simulink model "rct_CSTR_OL"  (R2022a)
settings: Solver=ode45  StartTime=0  StopTime=10  RelTol=1e-3  EnableMultiTasking=on
settings Model: Creator=The MathWorks, Inc.  LastModifiedBy=The MathWorks, Inc.
settings SolverCC: AlgebraicLoopSolver=TrustRegion  MaxZcPerStep=1
settings DataIOCC: InitialState=[311.267; 8.5695]  LimitDataPoints=on  SaveFormat=Array  ReturnWorkspaceOutputs=off  SignalLoggingName=logsOut
settings OptimizationCC: BooleanDataType=off  DefaultParameterBehavior=Inlined  InlineInvariantSignals=on  BufferReuse=off  ExpressionDepthLimit=2147483647  InitFltsAndDblsToZero=on  LifeSpan=inf
settings DebuggingCC: SaveWithParameterizedLinksMsg=none  UnderspecifiedInitializationDetection=Classic  MergeDetectMultiDrivingBlocksExec=none  CheckExecutionContextPreStartOutputMsg=on  SignalResolutionControl=TryResolveAllWithWarning  MultiTaskDSMMsg=warning  MultiTaskCondExecSysMsg=none  UnconnectedInputMsg=warning  UnconnectedOutputMsg=warning  UnconnectedLineMsg=warning  StateNameClashWarn=warning  SFUnexpectedBacktrackingDiag=warning  SFNoUnconditionalDefaultTransitionDiag=warning  SFExecutionAtInitializationDiag=none  SFMachineParentedDataDiag=warning  ArithmeticOperatorsInVariantConditions=warning
settings HardwareCC: ProdBitPerPointer=32  ProdBitPerSizeT=32  ProdBitPerPtrDiffT=32  ProdLargestAtomicFloat=None  ProdIntDivRoundTo=Undefined  ProdEndianess=Unspecified  ProdWordSize=32  ProdHWDeviceType=32-bit Generic  TargetUnknown=on
settings ModelReferenceCC: PropagateSignalLabelsOutOfModel=off
settings SFSimCC: SimUseLocalCustomCode=off  CustomCodeUndefinedFunction=UseInterfaceOnly
settings RTWCC: RTWUseLocalCustomCode=off  DLArmComputeVersion=19.05
settings CodeAppCC: StateflowObjectComments=on
settings GRTTargetCC: TargetFcnLib=ansi_tfl_tmw.mat  TargetLangStandard=C89/C90 (ANSI)  CombineOutputUpdateFcns=off  GRTInterface=on
settings ConfigComp: CovMetricSettings=dw  CovSaveCumulativeToWorkspaceVar=on  CovSaveSingleToWorkspaceVar=on  CovExternalEMLEnable=off

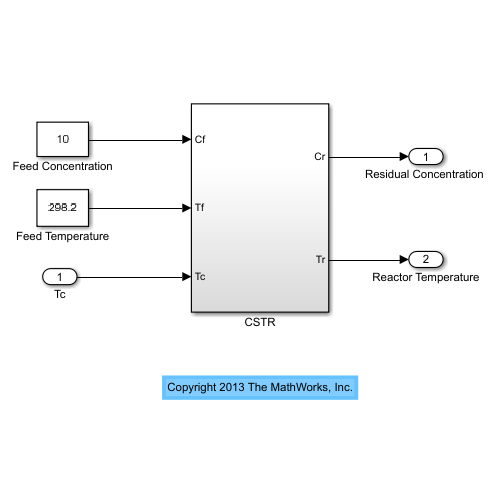
[thumbnail: Simulink's stored preview of the top-level diagram]
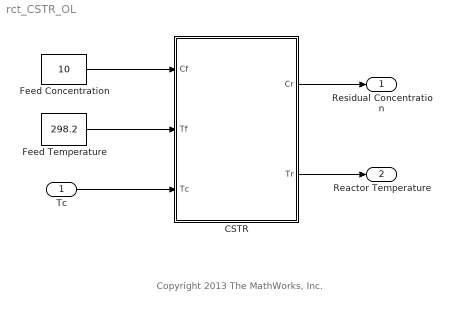
== system rct_CSTR_OL ==
  note: Copyright 2013 The MathWorks, Inc.
  Tc : Inport
  CSTR : Subsystem
  Feed Concentration : Constant  Value=10  SampleTime=0
  Feed Temperature : Constant  Value=298.2  SampleTime=0
  "Residual Concentration " : Outport
  Reactor Temperature : Outport  Port=2
  wires:
  Feed Concentration/1 -> CSTR/1(Cf)
  Feed Temperature/1 -> CSTR/2(Tf)
  CSTR/1(Cr) -> "Residual Concentration "/1
  CSTR/2(Tr) -> Reactor Temperature/1
  Tc/1 -> CSTR/3(Tc)

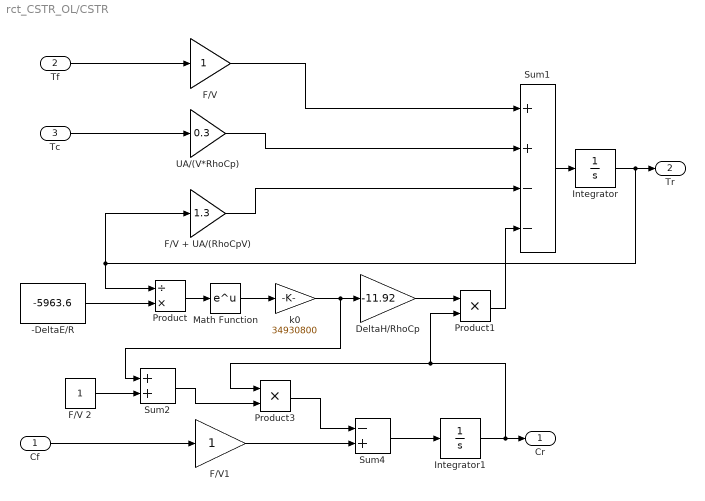
== system rct_CSTR_OL/CSTR ==
  Cf : Inport
  Tf : Inport  Port=2
  Tc : Inport  Port=3
  -DeltaE/R : Constant  Value=-5963.6  SampleTime=0
  DeltaH/RhoCp : Gain  Gain=-11.92  SaturateOnIntegerOverflow=on  OutDataTypeStr=Inherit: Same as input  ParamDataTypeStr=Inherit: Same as input
  F/V : Gain  SaturateOnIntegerOverflow=on  OutDataTypeStr=Inherit: Same as input  ParamDataTypeStr=Inherit: Same as input
  F/V + UA/(RhoCpV) : Gain  Gain=1.3  SaturateOnIntegerOverflow=on  OutDataTypeStr=Inherit: Same as input  ParamDataTypeStr=Inherit: Same as input
  F/V 2 : Constant  SampleTime=0
  F/V1 : Gain  SaturateOnIntegerOverflow=on  OutDataTypeStr=Inherit: Same as input  ParamDataTypeStr=Inherit: Same as input
  Integrator : Integrator  InitialCondition=311.26  LimitOutput=on  LowerSaturationLimit=0
  Integrator1 : Integrator  InitialCondition=8.57  LimitOutput=on  LowerSaturationLimit=0
  Math Function : Math  SignedPower=on
  Product : Product  Inputs=/*  InputSameDT=on  RndMeth=Zero  SaturateOnIntegerOverflow=on  OutDataTypeStr=Inherit: Same as first input
  Product1 : Product  InputSameDT=on  RndMeth=Zero  SaturateOnIntegerOverflow=on  OutDataTypeStr=Inherit: Same as first input
  Product3 : Product  InputSameDT=on  RndMeth=Zero  SaturateOnIntegerOverflow=on  OutDataTypeStr=Inherit: Same as first input
  Sum1 : Sum  Inputs=++--  InputSameDT=on  SaturateOnIntegerOverflow=on  OutDataTypeStr=Inherit: Same as first input
  Sum2 : Sum  InputSameDT=on  SaturateOnIntegerOverflow=on  OutDataTypeStr=Inherit: Same as first input
  Sum4 : Sum  Inputs=-+  InputSameDT=on  SaturateOnIntegerOverflow=on  OutDataTypeStr=Inherit: Same as first input
  UA/(V*RhoCp) : Gain  Gain=0.3  SaturateOnIntegerOverflow=on  OutDataTypeStr=Inherit: Same as input  ParamDataTypeStr=Inherit: Same as input
  k0 : Gain  Gain=34930800  SaturateOnIntegerOverflow=on  OutDataTypeStr=Inherit: Same as input  ParamDataTypeStr=Inherit: Same as input
  Cr : Outport
  Tr : Outport  Port=2
  wires:
  F/V/1 -> Sum1/1
  Sum1/1 -> Integrator/1
  Integrator/1 -> Product/1, F/V + UA/(RhoCpV)/1, Tr/1
  UA/(V*RhoCp)/1 -> Sum1/2
  F/V + UA/(RhoCpV)/1 -> Sum1/3
  Product/1 -> Math Function/1
  Math Function/1 -> k0/1
  DeltaH/RhoCp/1 -> Product1/1
  Product1/1 -> Sum1/4
  k0/1 -> DeltaH/RhoCp/1, Sum2/1
  -DeltaE/R/1 -> Product/2
  Product3/1 -> Sum4/1
  Sum4/1 -> Integrator1/1
  Integrator1/1 -> Product1/2, Product3/1, Cr/1
  F/V 2/1 -> Sum2/2
  F/V1/1 -> Sum4/2
  Tf/1 -> F/V/1
  Cf/1 -> F/V1/1
  Tc/1 -> UA/(V*RhoCp)/1
  Sum2/1 -> Product3/2
